simulink model "simulate_battery"  (R2021a)
settings: Solver=VariableStepAuto  StartTime=0.0  StopTime=time_val  RelTol=1e-3
settings Model: Creator=saleh  LastModifiedBy=saleh

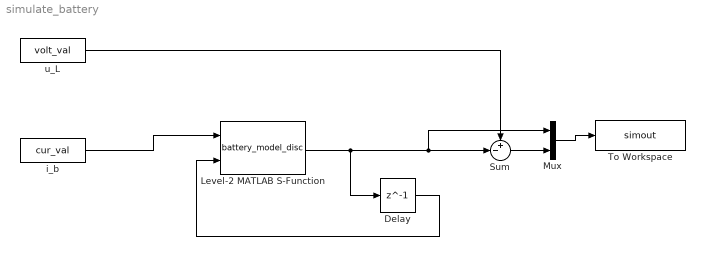
== system simulate_battery ==
  Delay : Delay  DelayLength=1  InitialCondition=volt_est.Data(end)
  Level-2 MATLAB S-Function : M-S-Function  FunctionName=battery_model_disc  Parameters=Delta, x_conv, Qe, Cg
  Mux : Mux  Inputs=2
  Sum : Sum  Inputs=+-|
  To Workspace : ToWorkspace  VariableName=simout  SaveFormat=Timeseries  SampleTime=-1
  i_b : FromWorkspace  VariableName=cur_val
  u_L : FromWorkspace  VariableName=volt_val
  wires:
  Level-2 MATLAB S-Function/1 -> Mux/1, Sum/2, Delay/1
  u_L/1 -> Sum/1
  i_b/1 -> Level-2 MATLAB S-Function/1
  Delay/1 -> Level-2 MATLAB S-Function/2
  Sum/1 -> Mux/2
  Mux/1 -> To Workspace/1
